simulink model "pid_exp"  (R2024b)
settings: Solver=FixedStepAuto  StartTime=0.0  StopTime=simTime  FixedStep=0.1  RelTol=1e-3  EnableMultiTasking=on
values from neighbouring files (symbols this model uses):
  setpoint = str2double(get(editSetpoint, 'String'))    [gui_pid_simulation_2.m]
undefined symbols (not defined in the file or in its folder): kd, ki, kp, m_on
libraries: arduinolib x3, dspfdesign x1, dspstat3 x1, arduinosensorlib x1
settings Model: SimulationMode=external  ExtModeTrigDuration=2  Creator=labadmin  LastModifiedBy=labadmin
settings SolverCC: AutoInsertRateTranBlk=on
settings OptimizationCC: EnhancedBackFolding=on  PassReuseOutputArgsAs=Individual arguments  ZeroExternalMemoryAtStartup=off  ZeroInternalMemoryAtStartup=off  MaxStackSize=64  OptimizeBlockOrder=speed  DifferentSizesBufferReuse=on  OptimizationCustomize=off  EfficientTunableParamExpr=on
settings DebuggingCC: ParameterTunabilityLossMsg=error
settings HardwareCC: ProdBitPerPointer=32  ProdBitPerSizeT=32  ProdBitPerPtrDiffT=32  ProdLargestAtomicInteger=Long  ProdLargestAtomicFloat=Double  ProdWordSize=32  ProdHWDeviceType=ARM Compatible->ARM Cortex  UseEmbeddedCoderFeatures=off  UseSimulinkCoderFeatures=off
settings SFSimCC: MATLABDynamicMemAlloc=off
settings RTWCC: Description=Embedded Coder  SystemTargetFile=ert.tlc  HardwareBoard=Arduino Uno R4 WiFi  TemplateMakefile=ert_default_tmf  Toolchain=Arduino ARM M4  BuildConfiguration=Faster Runs
settings CodeAppCC: ForceParamTrailComments=on  IgnoreCustomStorageClasses=off  OperatorAnnotations=on  SimulinkDataObjDesc=on  SFDataObjDesc=on  MangleLength=10  InsertBlockDesc=on
settings ERTTargetCC: SupportContinuousTime=on  SupportNonInlinedSFcns=on  SupportVariableSizeSignals=on  ExtModeTransport=3  ExtModeStaticAlloc=on  ExtModeAutomaticAllocSize=off  ExtModeStaticAllocSize=8192  ExtModeMexFile=ext_xcp  ExtModeIntrfLevel=Level2 - Open  InlinedParameterPlacement=Hierarchical

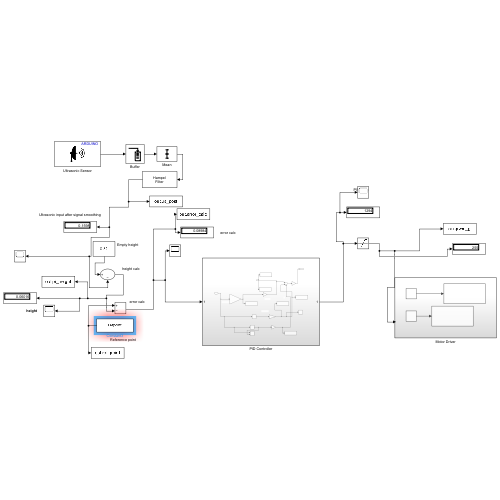
[thumbnail: Simulink's stored preview of the top-level diagram]
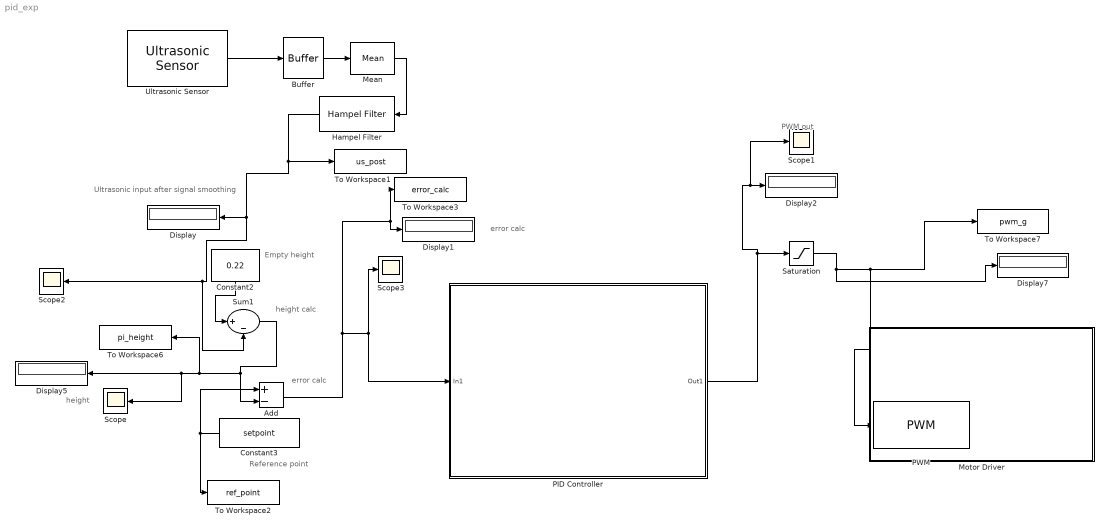
== system pid_exp ==
  note: Empty height
  note: height calc
  note: error calc
  note: height
  note: PWM out
  note: Ultrasonic input after signal smoothing
  note: error calc
  note: Reference point
  Add : Sum  Inputs=+-
  Buffer : Buffer  N=5  OutputFrames=off
  Constant2 : Constant  Value=0.22
  Constant3 : Constant  Value=setpoint
  Display{,1..2,5,7} (5 alike) : Display
  Hampel Filter : dspfdesign/Hampel Filter  WindowLength=5  ThresholdPort=off  Threshold=3  EnableIsOutlierOutput=off  SimulateUsing=Interpreted execution
  Mean : dspstat3/Mean  run=off  InputProcessing=Columns as channels (frame based)  reset_popup=None  directionMode=Each column  dimension=1  roiEnable=off  roiType=Rectangles  roiPortion=Entire ROI  roiOutput=Individual statistics for each ROI  roiFlag=off  roundingMode=Floor  overflowMode=off  outputDataTypeStr=Inherit: Same as accumulator  outputMin=[]  outputMax=[]  outputLastDataTypeStr=Inherit: Same as accumulator
  Motor Driver : Subsystem
  PID Controller : Subsystem
  PWM : arduinolib/PWM  pinNumber=6  frequencyType=Default  desiredFrequency=490.2  achievableFrequency=490.2
  Saturation : Saturate  UpperLimit=255  LowerLimit=0
  Scope{,1..3} (4 alike) : Scope
  Sum1 : Sum  Inputs=|+-
  To Workspace1 : ToWorkspace  VariableName=us_post  SaveFormat=Timeseries  SampleTime=-1
  To Workspace2 : ToWorkspace  VariableName=ref_point  SaveFormat=Timeseries  SampleTime=-1
  To Workspace3 : ToWorkspace  VariableName=error_calc  SaveFormat=Timeseries  SampleTime=-1
  To Workspace6 : ToWorkspace  VariableName=pi_height  SaveFormat=Timeseries  SampleTime=-1
  To Workspace7 : ToWorkspace  VariableName=pwm_g  SaveFormat=Timeseries  SampleTime=-1
  Ultrasonic Sensor : arduinosensorlib/Ultrasonic Sensor  NumSignalPins=2  TrigPin=2  EchoPin=3  SignalPin=3  SampleTime_=0.1  blockPlatform=ARDUINO
  wires:
  Constant2/1 -> Sum1/1
  Mean/1 -> Hampel Filter/1
  Sum1/1 -> To Workspace6/1, Scope/1, Display5/1, Add/2
  Constant3/1 -> To Workspace2/1, Add/1
  Ultrasonic Sensor/1 -> Buffer/1
  Add/1 -> To Workspace3/1, Display1/1, PID Controller/1(In1), Scope3/1
  Buffer/1 -> Mean/1
  Saturation/1 -> PWM/1, To Workspace7/1, Display7/1
  Hampel Filter/1 -> Display/1, Sum1/2, Scope2/1, To Workspace1/1
  PID Controller/1(Out1) -> Scope1/1, Display2/1, Saturation/1

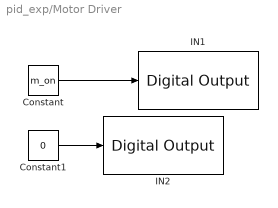
== system pid_exp/Motor Driver ==
  Constant : Constant  Value=m_on
  Constant1 : Constant  Value=0
  IN1 : arduinolib/Digital Output  pinNumber=10  Direction=output  blockPlatform=arduino
  IN2 : arduinolib/Digital Output  pinNumber=11  Direction=output  blockPlatform=arduino
  wires:
  Constant/1 -> IN1/1
  Constant1/1 -> IN2/1

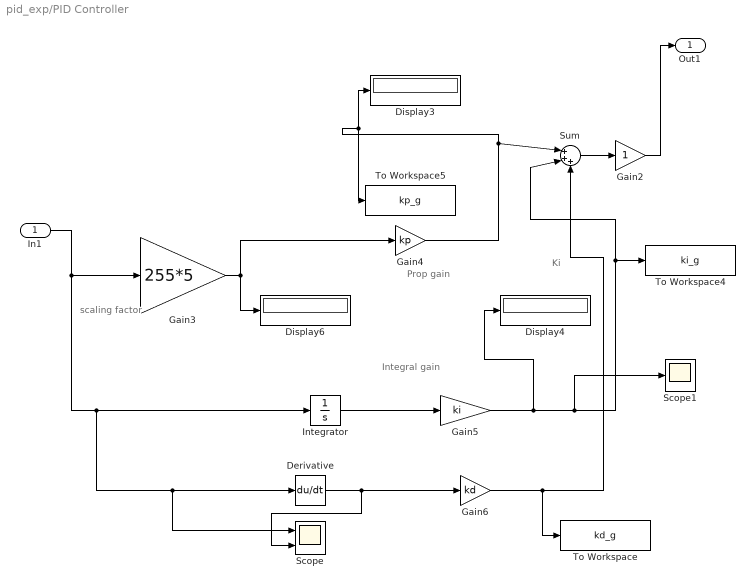
== system pid_exp/PID Controller ==
  note: scaling factor
  note: Integral gain
  note: Ki
  note: Prop gain
  In1 : Inport
  Derivative : Derivative
  Display3 : Display
  Display4 : Display
  Display6 : Display
  Gain2 : Gain
  Gain3 : Gain  Gain=255*5
  Gain4 : Gain  Gain=kp
  Gain5 : Gain  Gain=ki
  Gain6 : Gain  Gain=kd
  Integrator : Integrator
  Scope : Scope  NumInputPorts=2
  Scope1 : Scope
  Sum : Sum  Inputs=|+++
  To Workspace : ToWorkspace  VariableName=kd_g  SaveFormat=Timeseries  SampleTime=-1
  To Workspace4 : ToWorkspace  VariableName=ki_g  SaveFormat=Timeseries  SampleTime=-1
  To Workspace5 : ToWorkspace  VariableName=kp_g  SaveFormat=Timeseries  SampleTime=-1
  Out1 : Outport
  wires:
  Gain6/1 -> To Workspace/1, Sum/3
  Derivative/1 -> Scope/2, Gain6/1
  Integrator/1 -> Gain5/1
  Sum/1 -> Gain2/1
  Gain2/1 -> Out1/1
  Gain5/1 -> Display4/1, Scope1/1, Sum/2, To Workspace4/1
  Gain4/1 -> Display3/1, To Workspace5/1, Sum/1
  In1/1 -> Scope/1, Derivative/1, Integrator/1, Gain3/1
  Gain3/1 -> Gain4/1, Display6/1
